simulink model "Automata"  (R2018a)
settings: Solver=VariableStepAuto  StartTime=0.0  StopTime=inf  FixedStep=0.001  RelTol=1e-3
values from neighbouring files (symbols this model uses):
  bcx = 1000e3    (= 1000000)    [Variables.m]
  bcy = 500e3    (= 500000)    [Variables.m]
  beq1 = 30    [Variables.m]
  beq2 = 18    [Variables.m]
  bw = 30000    [Variables.m]
  g = 9.81    [Variables.m]
  Jeq1 = Jwc+Jmc*(rc^2)    (= 2252)    [Variables.m]
  Jeq2 = Jd+Jmi*(riz^2)    (= 27008)    [Variables.m]
  kcy = 1.3e11    (= 130000000000)    [Variables.m]
  Kw = 1800e3    (= 1800000)    [Variables.m]
  Mc = 50000    [Variables.m]
  Mt = Mc+Jeq1*(1/(Rw^2))    (= 59008)    [Variables.m]
  rc = 15    [Variables.m]
  Rd = 0.75    [Variables.m]
  riz = 30    [Variables.m]
  Rw = 0.5    [Variables.m]
  Y_t0 = 45    [Variables.m]
undefined symbols (not defined in the file or in its folder): AlturaInicialBarco, AlturaInicialMuelle, cont_muelle_masa, contenedores, PObjetivo_fijo, PObjetivo_incremental, x_der, x_izq, Y_inf_barco, Y_max, Y_muelle, Y_sb
settings Model: Creator=lauta  LastModifiedBy=lauta
settings SolverCC: AlgebraicLoopSolver=LineSearch

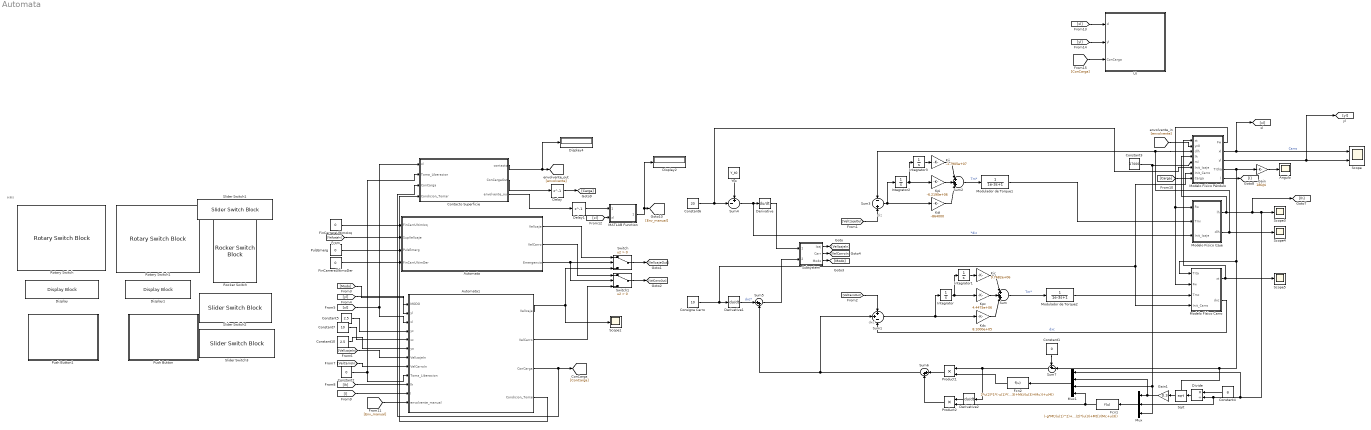
== system Automata ==
  note: HMI
  note: diz
  note: dxc
  Angulo : Scope
  Automata : Stateflow chart  TreatAsAtomicUnit=on
  Automata1 : Stateflow chart  TreatAsAtomicUnit=on
  Consigna Carro : Constant  Value=10
  Constant1 : Constant  Value=0
  Constant10 : Constant  Value=2.5
  Constant2 : Constant  Value=0
  Constant3 : Constant  Value=17000
  Constant4 : Constant  Value=g
  Constant5 : Constant  Value=2.5
  Constant6 : Constant  Value=20
  Constant7 : Constant  Value=10
  Contacto Superficie : Stateflow chart  TreatAsAtomicUnit=on
  Delay : Delay  DelayLength=1  InitialCondition=0
  Delay1 : Delay  DelayLength=1  InitialCondition=0
  Derivative : Derivative
  Derivative1 : Derivative
  Derivative2 : Derivative
  Display : DisplayBlock  WebBlockId=717  LabelPosition=Hide
  Display1 : DisplayBlock  WebBlockId=718  LabelPosition=Hide
  Display2 : Display
  Display4 : Display
  Divide : Product  Inputs=*/
  Fcn1 : Fcn  Expr=(-g*Mt/(u(1)^2)+u(2)*(u(3)+Mt))/(Mc+u(3))
  Fcn2 : Fcn  Expr=2*u(2)*1*(-u(1)*((u(3)+Mt)/(u(3)+Mc))+u(4))
  FinCarreraUltimoDer : Constant  Value=0
  FinCarreraUltimoIzq : Constant  Value=0
  Gain : Gain  Gain=180/pi
  Gain1 : Gain  Gain=0.3
  Integrator{,1..3} (4 alike) : Integrator
  Kdc : Gain  Gain=8.1000e+05
  Kdi : Gain  Gain=-864000
  Kic : Gain  Gain=9.7682e+06
  Kii : Gain  Gain=-1.7905e+07
  Kpc : Gain  Gain=4.4475e+06
  Kpi : Gain  Gain=-6.2190e+06
  MATLAB Function : MATLAB Function  TreatAsAtomicUnit=on
  "Modelo Físico Carro " : Subsystem
  Modelo Físico Izaje : Subsystem
  "Modelo Físico Péndulo " : Subsystem
  Modulador de Torque1 : TransferFcn  Denominator=[1e-3 1]
  Modulador de Torque2 : TransferFcn  Denominator=[1e-3 1]
  Mux : Mux  Inputs=3
  Mux1 : Mux
  Product1 : Product
  Product2 : Product
  PulsEmerg : Constant  Value=0
  Push Button : Subsystem  DialogController=hmiCreateDDGDialog  IsWebBlock=on  mask(MWDashboardBlock){webBlockId=2acad30b-f587-4c91-b113-839cda201c99, webBlockType=pushbutton, ShowInLibBrwoser=on, ShowInitialText=on, HMISrcModelName=Automata}
      mask prompts: webBlockId "WebBlock Id"; webBlockType "WebBlock Type"; HMISrcModelName "Source Model"
      mask help: SimulinkHMI:dialogs:PushButtonDialogDesc
      mask Help: helpview([docroot '/mapfiles/simulink.map'], 'hmi_push_button')
      mask Display:
      | model = bdroot(gcb);
      | if strcmp(get_param(model,'BlockDiagramType'), 'library')
      |     image([(matlabroot) '/toolbox/simulink/hmi/icons/PushButton.png']);
      | end
  Push Button1 : Subsystem  DialogController=hmiCreateDDGDialog  IsWebBlock=on  mask(MWDashboardBlock){webBlockId=d4af1492-9a98-42f0-a069-3443a3c3e2ec, webBlockType=pushbutton, ShowInLibBrwoser=on, ShowInitialText=on, HMISrcModelName=Automata}
      mask prompts: webBlockId "WebBlock Id"; webBlockType "WebBlock Type"; HMISrcModelName "Source Model"
      mask help: SimulinkHMI:dialogs:PushButtonDialogDesc
      mask Help: helpview([docroot '/mapfiles/simulink.map'], 'hmi_push_button')
      mask Display:
      | model = bdroot(gcb);
      | if strcmp(get_param(model,'BlockDiagramType'), 'library')
      |     image([(matlabroot) '/toolbox/simulink/hmi/icons/PushButton.png']);
      | end
  Rocker Switch : RockerSwitchBlock  WebBlockId=682  LabelPosition=Hide
      settings: Values={{'Automatico', 'Manual'}, [-1 1]}
  Rotary Switch : RotarySwitchBlock  WebBlockId=715
      settings: Values={{'High', 'Medium', 'Low', 'OFF', 'Low', 'Medium', 'High'}, [-0.15 -0.05 -0.01 0 0.01 0.05 0.15]}
  Rotary Switch1 : RotarySwitchBlock  WebBlockId=716
      settings: Values={{'High', 'Medium', 'Low', 'OFF', 'Low', 'Medium', 'High'}, [-0.15 -0.05 -0.01 0 0.01 0.05 0.15]}
  Scope : Scope  NumInputPorts=2
  Scope{1,3..5} (4 alike) : Scope
  Slider Switch1 : SliderSwitchBlock  WebBlockId=725
      settings: Values={{'OK', 'STOP'}, [0 1]}
  Slider Switch2 : SliderSwitchBlock  WebBlockId=741
      settings: Values={{'OK', 'LimDerecho'}, [0 1]}
  Slider Switch3 : SliderSwitchBlock  WebBlockId=742
      settings: Values={{'OK', 'LimIzquierdo'}, [0 1]}
  Sqrt : Sqrt  SaturateOnIntegerOverflow=on
  Subsystem : Subsystem
  Sum : Sum  Inputs=|+++|
  Sum1 : Sum  Inputs=++-
  Sum2 : Sum  Inputs=|+++|
  Sum3 : Sum  Inputs=-+
  Sum4 : Sum  Inputs=+-|
  Sum5 : Sum  Inputs=|++
  Sum6 : Sum  Inputs=|++
  Sum7 : Sum  Inputs=+-|
  Switch : Switch  Criteria=u2 > Threshold
  Switch1 : Switch  Criteria=u2 > Threshold
  UI : Stateflow chart  TreatAsAtomicUnit=on
  Yto : Constant  Value=Y_t0
  wires:
  Modelo Físico Izaje/1(lh) -> [lh], Scope3/1, Mux1/1, Divide/2, Mux/2, "Modelo Físico Péndulo "/4(lh)
  Modelo Físico Izaje/2(dlh) -> Scope4/1, "Modelo Físico Péndulo "/3(dlh), Sum3/1
  "Modelo Físico Carro "/1(xt) -> "Modelo Físico Péndulo "/1(xt), Scope5/1
  "Modelo Físico Péndulo "/1(Fw) -> "Modelo Físico Carro "/2(Fw), Modelo Físico Izaje/1(Fw)
  "Modelo Físico Péndulo "/2(xl) -> [xl], Scope/1  "Carro"
  Kpc/1 -> Sum/2
  Sum1/1 -> Kdc/1, Integrator/1
  Integrator/1 -> Kpc/1, Integrator1/1
  Sum/1 -> Modulador de Torque2/1  "Tm*"
  Kdc/1 -> Sum/3
  Integrator1/1 -> Kic/1
  Kic/1 -> Sum/1
  Kii/1 -> Sum2/1
  Integrator3/1 -> Kii/1
  Sum2/1 -> Modulador de Torque1/1  "Tm*"
  Sum3/1 -> Kdi/1, Integrator2/1
  Kdi/1 -> Sum2/3
  Integrator2/1 -> Integrator3/1, Kpi/1
  Kpi/1 -> Sum2/2
  Gain/1 -> Angulo/1
  "Modelo Físico Péndulo "/4(Titha) -> "Modelo Físico Carro "/1(Tita), Sum7/2, Gain/1
  "Modelo Físico Carro "/2(dxc) -> Sum1/3  "dxc"
  Constant3/1 -> Mux/3, Mux1/3, "Modelo Físico Péndulo "/5(ml)
  Modulador de Torque1/1 -> Modelo Físico Izaje/2(Tmi)
  Product1/1 -> Sum6/1
  Product2/1 -> Sum6/2
  Fcn2/1 -> Product1/2
  Fcn1/1 -> Mux1/4, Product2/2
  Sum7/1 -> Product1/1, Derivative2/1
  Derivative2/1 -> Product2/1
  Divide/1 -> Sqrt/1
  Constant4/1 -> Divide/1
  Sqrt/1 -> Gain1/1
  Mux/1 -> Fcn1/1
  Gain1/1 -> Mux1/2, Mux/1
  Mux1/1 -> Fcn2/1
  Constant1/1 -> Sum7/1
  Modulador de Torque2/1 -> "Modelo Físico Carro "/3(Tmc)
  Sum4/1 -> Modelo Físico Izaje/3(Init_Izaje), Derivative/1  "*diz"
  Sum6/1 -> Sum1/2, Sum5/2
  Constant6/1 -> "Modelo Físico Péndulo "/6(Init_Izaje), Sum4/2
  Yto/1 -> Sum4/1
  Consigna Carro/1 -> "Modelo Físico Péndulo "/7(Init_Carro), "Modelo Físico Carro "/4(Init_Carro), Derivative1/1
  Derivative/1 -> Subsystem/1(VelIzaje)
  Derivative1/1 -> Sum5/1  "dxc*"
  Sum5/1 -> Subsystem/2(VelCarro)
  FinCarreraUltimoIzq/1 -> Automata/1(FinCarrUltimIzq)
  [VelIzajeIn] -> Automata/2(SupVelIzaje)
  PulsEmerg/1 -> Automata/3(PulsEmerg)
  FinCarreraUltimoDer/1 -> Automata/4(FinCarrUltimDer)
  Automata/3(Emergencia) -> Switch1/2, Switch/2
  Automata1/1(VelIzaje) -> Scope1/1, Switch/3
  Automata/1(VelIzaje) -> Switch/1
  Automata1/2(VelCarro) -> Switch1/3
  Automata/2(VelCarro) -> Switch1/1
  Subsystem/1(Izaj) -> [VelIzajeIn]
  Switch/1 -> [VelIzajeOut]
  [VelIzajeOut] -> Sum3/2
  [VelCarroOut] -> Sum1/1
  Switch1/1 -> [VelCarroOut]
  Subsystem/3(Modo) -> [Modo]
  [Modo] -> Automata1/1(MODO)
  Subsystem/2(Carr) -> [VelCarroIn]
  [yl] -> Automata1/2(yl)
  [xl] -> Automata1/3(xl), Contacto Superficie/1(xl)
  [VelIzajeIn] -> Automata1/7(VelIzajeIn)
  [VelCarroIn] -> Automata1/8(VelCarroIn)
  Constant2/1 -> Contacto Superficie/2(Toma_Liberacion), Automata1/9(Toma_Liberacion)
  "Modelo Físico Péndulo "/5(l) -> [l]
  [lh] -> Automata1/10(lh)
  [l] -> Automata1/11(l)
  Constant7/1 -> Automata1/5(xc)
  Constant5/1 -> Automata1/4(yc)
  Constant10/1 -> Automata1/6(yo)
  [envolvente] -> "Modelo Físico Péndulo "/2(yc0)
  Automata1/3(ConCarga) -> [ConCarga], Contacto Superficie/3(ConCarga)
  "Modelo Físico Péndulo "/3(yl) -> [yl], Scope/2
  [Carga] -> "Modelo Físico Péndulo "/8(Carga)
  Contacto Superficie/1(contacto) -> Display4/1, [envolvente]
  Contacto Superficie/2(ConCargaOut) -> Delay/1
  Delay/1 -> [Carga]
  Automata1/4(Condicion_Tomar) -> Contacto Superficie/4(Condicion_Tomar)
  Contacto Superficie/3(envolvente_out) -> Delay1/1
  MATLAB Function/1(altura_manual) -> Display2/1, [Env_manual]
  [Env_manual] -> Automata1/12(envolvente_manual)
  Delay1/1 -> MATLAB Function/1(envolventes)
  [xl] -> MATLAB Function/2(xl)
  [xl] -> UI/1(xl)
  [yl] -> UI/2(yl)
  [ConCarga] -> UI/3(ConCarga)

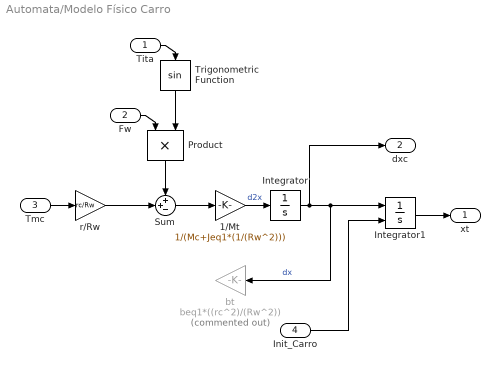
== system Automata/Modelo Físico Carro  ==
  Tita : Inport
  Fw : Inport  Port=2
  Tmc : Inport  Port=3
  Init_Carro : Inport  Port=4
  1/Mt : Gain  Gain=1/(Mc+Jeq1*(1/(Rw^2)))
  Integrator : Integrator
  Integrator1 : Integrator  InitialConditionSource=external
  Product : Product
  Sum : Sum  Inputs=++-
  Trigonometric Function : Trigonometry
  bt : Gain  Commented=on  Gain=beq1*((rc^2)/(Rw^2))
  "r/Rw " : Gain  Gain=rc/Rw
  xt : Outport
  dxc : Outport  Port=2
  wires:
  Tita/1 -> Trigonometric Function/1
  Integrator/1 -> dxc/1, bt/1, Integrator1/1  "dx"
  Product/1 -> Sum/1
  "r/Rw "/1 -> Sum/2
  Sum/1 -> 1/Mt/1
  Trigonometric Function/1 -> Product/2
  Integrator1/1 -> xt/1
  1/Mt/1 -> Integrator/1  "d2x"
  Tmc/1 -> "r/Rw "/1
  Fw/1 -> Product/1
  Init_Carro/1 -> Integrator1/2

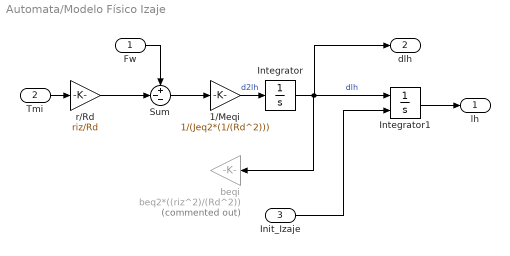
== system Automata/Modelo Físico Izaje ==
  Fw : Inport
  Tmi : Inport  Port=2
  Init_Izaje : Inport  Port=3
  1/Meqi : Gain  Gain=1/(Jeq2*(1/(Rd^2)))
  Integrator : Integrator
  Integrator1 : Integrator  InitialConditionSource=external
  Sum : Sum  Inputs=+--
  beqi : Gain  Commented=on  Gain=beq2*((riz^2)/(Rd^2))
  "r/Rd " : Gain  Gain=riz/Rd
  lh : Outport
  dlh : Outport  Port=2
  wires:
  "r/Rd "/1 -> Sum/2
  Sum/1 -> 1/Meqi/1
  Integrator/1 -> beqi/1, dlh/1, Integrator1/1  "dlh"
  Tmi/1 -> "r/Rd "/1
  Integrator1/1 -> lh/1
  1/Meqi/1 -> Integrator/1  "d2lh"
  Fw/1 -> Sum/1
  Init_Izaje/1 -> Integrator1/2

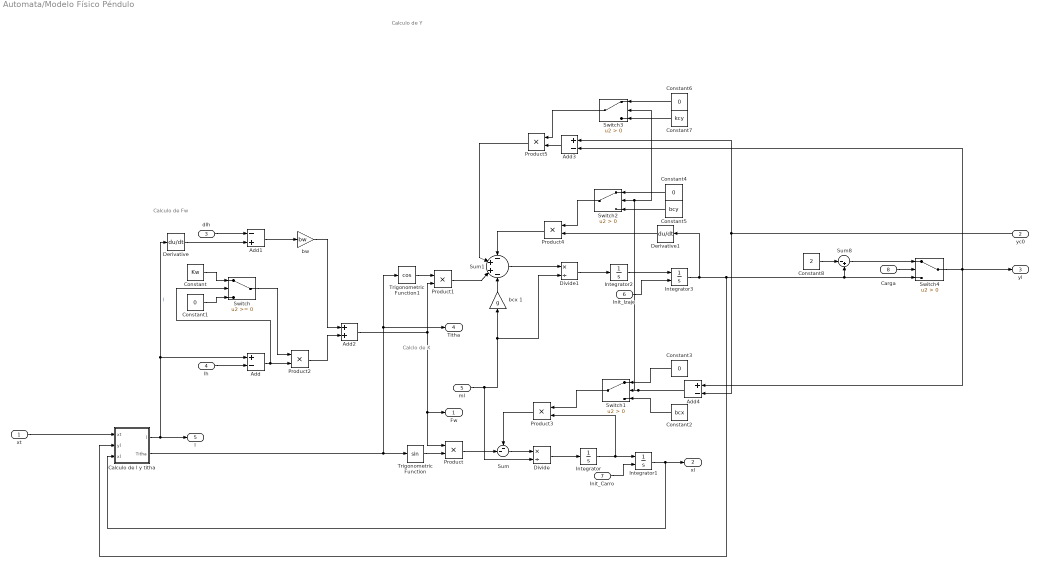
== system Automata/Modelo Físico Péndulo  ==
  note: Calculo de Fw
  note: Calclo de X
  note: Calculo de Y
  xt : Inport
  yc0 : Inport  Port=2
  dlh : Inport  Port=3
  lh : Inport  Port=4
  ml : Inport  Port=5
  Init_Izaje : Inport  Port=6
  Init_Carro : Inport  Port=7
  Carga : Inport  Port=8
  Add : Sum  Inputs=+-
  Add1 : Sum  Inputs=-+
  Add2 : Sum
  Add3 : Sum  Inputs=+-
  Add4 : Sum  Inputs=+-
  Calculo de l y titha : Subsystem
  Constant : Constant  Value=Kw
  Constant{1,3..4,6} (4 alike) : Constant  Value=0
  Constant2 : Constant  Value=bcx
  Constant5 : Constant  Value=bcy
  Constant7 : Constant  Value=kcy
  Constant8 : Constant  Value=2
  Derivative : Derivative
  Derivative1 : Derivative
  Divide : Product  Inputs=*/
  Divide1 : Product  Inputs=*/
  Integrator : Integrator
  Integrator1 : Integrator  InitialConditionSource=external
  Integrator2 : Integrator
  Integrator3 : Integrator  InitialConditionSource=external  InitialCondition=20
  Product{,1..5} (6 alike) : Product
  Sum : Sum  Inputs=--|
  Sum1 : Sum  Inputs=-|+|+|-
  Sum8 : Sum  Inputs=|-+
  Switch : Switch
  Switch{1..4} (4 alike) : Switch  Criteria=u2 > Threshold
  Trigonometric Function : Trigonometry
  Trigonometric Function1 : Trigonometry  Operator=cos
  bcx 1 : Gain  Gain=g
  bw : Gain  Gain=bw
  Fw : Outport
  xl : Outport  Port=2
  yl : Outport  Port=3
  Titha : Outport  Port=4
  l : Outport  Port=5
  wires:
  xt/1 -> Calculo de l y titha/1(xt)
  Calculo de l y titha/1(l) -> Add/1, Derivative/1, l/1  "l"
  lh/1 -> Add/2
  Add/1 -> Switch/2, Product2/2
  Add1/1 -> bw/1
  Product2/1 -> Add2/2
  bw/1 -> Add2/1
  dlh/1 -> Add1/1
  Derivative/1 -> Add1/2
  Add2/1 -> Fw/1, Product/1, Product1/2
  Trigonometric Function/1 -> Product/2
  Calculo de l y titha/2(Titha) -> Titha/1, Trigonometric Function1/1, Trigonometric Function/1
  Product/1 -> Sum/2
  Sum/1 -> Divide/1
  Integrator/1 -> Product3/2, Integrator1/1
  Product3/1 -> Sum/1
  Integrator1/1 -> xl/1, Calculo de l y titha/3(xl)
  Trigonometric Function1/1 -> Product1/1
  ml/1 -> Divide1/2, bcx 1/1, Divide/2
  Divide/1 -> Integrator/1
  Product1/1 -> Sum1/3
  bcx 1/1 -> Sum1/4
  yc0/1 -> Add3/1, Add4/2
  Product5/1 -> Sum1/2
  Product4/1 -> Sum1/1
  Integrator2/1 -> Integrator3/1
  Sum1/1 -> Divide1/1
  Divide1/1 -> Integrator2/1
  Switch/1 -> Product2/1
  Constant/1 -> Switch/1
  Constant1/1 -> Switch/3
  Switch1/1 -> Product3/1
  Add4/1 -> Switch3/2, Switch2/2, Switch1/2
  Constant3/1 -> Switch1/1
  Constant2/1 -> Switch1/3
  Switch2/1 -> Product4/1
  Constant4/1 -> Switch2/1
  Constant5/1 -> Switch2/3
  Add3/1 -> Product5/2
  Switch3/1 -> Product5/1
  Constant6/1 -> Switch3/1
  Constant7/1 -> Switch3/3
  Derivative1/1 -> Product4/2
  Init_Carro/1 -> Integrator1/2
  Init_Izaje/1 -> Integrator3/2
  Switch4/1 -> Add3/2, Add4/1, yl/1
  Constant8/1 -> Sum8/1
  Sum8/1 -> Switch4/1
  Carga/1 -> Switch4/2
  Integrator3/1 -> Calculo de l y titha/2(yl), Switch4/3, Sum8/2, Derivative1/1

== system Automata/Push Button ==

== system Automata/Push Button1 ==

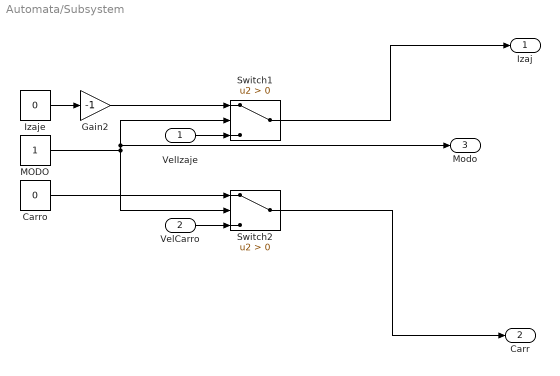
== system Automata/Subsystem ==
  VelIzaje : Inport
  VelCarro : Inport  Port=2
  Carro : Constant  Value=0
  Gain2 : Gain  Gain=-1
  Izaje : Constant  Value=0
  MODO : Constant
  Switch1 : Switch  Criteria=u2 > Threshold
  Switch2 : Switch  Criteria=u2 > Threshold
  Izaj : Outport
  Carr : Outport  Port=2
  Modo : Outport  Port=3
  wires:
  Gain2/1 -> Switch1/1
  Izaje/1 -> Gain2/1
  Switch1/1 -> Izaj/1
  MODO/1 -> Modo/1, Switch1/2, Switch2/2
  Carro/1 -> Switch2/1
  Switch2/1 -> Carr/1
  VelIzaje/1 -> Switch1/3
  VelCarro/1 -> Switch2/3

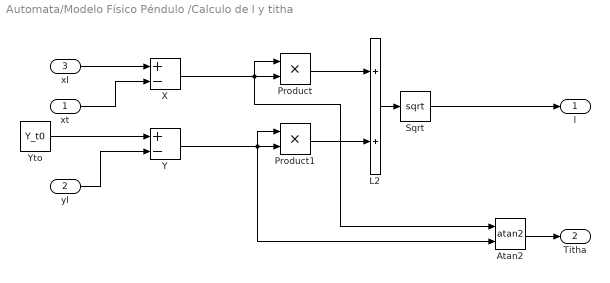
== system Automata/Modelo Físico Péndulo /Calculo de l y titha ==
  xt : Inport
  yl : Inport  Port=2
  xl : Inport  Port=3
  Atan2 : Trigonometry  Operator=atan2
  L2 : Sum
  Product : Product
  Product1 : Product
  Sqrt : Sqrt  SaturateOnIntegerOverflow=on
  X : Sum  Inputs=+-
  Y : Sum  Inputs=+-
  Yto : Constant  Value=Y_t0
  l : Outport
  Titha : Outport  Port=2
  wires:
  Y/1 -> Atan2/2, Product1/1, Product1/2
  X/1 -> Product/2, Atan2/1, Product/1
  Product1/1 -> L2/2
  L2/1 -> Sqrt/1
  yl/1 -> Y/2
  Product/1 -> L2/1
  Yto/1 -> Y/1
  xl/1 -> X/1
  Sqrt/1 -> l/1
  xt/1 -> X/2
  Atan2/1 -> Titha/1

== stateflow chart Automata/Automata ==
  state NIVEL_0
    if PulsEmerg==1 || FinCarrUltimDer==1 || FinCarrUltimIzq==1 || SupVelIzaje>10
    VelIzaje=0;
    VelCarro=0;
    Emergencia=1;
    else
    Emergencia=-1;
    end
  (default) -> NIVEL_0
  data: FinCarrUltimIzq input; SupVelIzaje input; PulsEmerg input; FinCarrUltimDer input; VelIzaje output; VelCarro output; Emergencia output

== stateflow chart Automata/Automata1 ==
  state NIVEL_1
    contenedores;
    cont_muelle_masa;
    entry: ConCarga=-1;
    note: -Comando operador
        | -Limites normales de oepracion
        | 	-Activacion/desactivacion de control de angulo
        | 	-Fines de carrera
        | 	-Control de Velocidad
        | 	-Estado de carga
        | 		-4 Sensores
        | 		-Twistlook
        | 	-Deteccion cable de izaje flojo
        | 	-Sensor de angulo
    state MODOS [parallel]
      settings: executionOrder=1
      state MANUAL
        state Liberacion
          Condicion_Tomar=-1;
          if Toma_Liberacion==-1
          ConCarga=-1;
          end
        state Toma
          Condicion_Tomar=1;
          if Toma_Liberacion==1
          ConCarga=1;
          end
        state Aproximacion
          Condicion_Tomar=0;
          VelCarro=VelCarroIn*0.1;
          VelIzaje=VelIzajeIn*0.1;
        note: -Falta asignar yc = y consigna
            | -Falta asignar xc = x consigna
        (junction 70) -> Toma [order 1] : [ConCarga==-1]
        (junction 70) -> Liberacion [order 2] : [ConCarga==1]
        Aproximacion -> (junction 70) : [yl==yc && xl<xc+0.1 && xl>xc-0.1]
        (default) -> Aproximacion
        Toma -> Aproximacion : [ConCarga==1]
        Liberacion -> Aproximacion : [ConCarga==-1]
      note: -Falta asignar yo como yc anterior
      state AUTOMATICO
        state CONFIGURACION
          x_izq;
          x_der;
          PObjetivo_incremental;
          PObjetivo_fijo;
          Y_inf_barco;
          Y_muelle;
          Y_t0;
          Y_max;
          Y_sb;
          AlturaInicialMuelle;
          AlturaInicialBarco;
        state CICLOS
          VelIzaje=VelIzajeIn;
          VelCarro=VelCarroIn;
          note: -Toma de carga (M) OK
              | -Izaje y traslacion (A)
              | -Parada y descenso (A)
              | -Aproximacion fina (M) OK
              | -Liberacion de carga (M) OK
              | -Retorno vacio (A)
        (default) -> CONFIGURACION
        CONFIGURACION -> CICLOS
      (default) -> MANUAL
      MANUAL -> AUTOMATICO : [((yl>(yo+2.5))  &&xl<0) || ((yl>(yo+2.5)) && xl>5)]
      AUTOMATICO -> MANUAL : [((yl<(yc+2.5) && xl<xc+0.1 && xl>xc-0.1) && xl<0) || ((yl<(yc+2.5) && xl<xc+0.1 && xl>xc-0.1) && xl>5)]
  (default) -> NIVEL_1
  data: VelIzaje output; VelCarro output; MODO input; yl input; Y_inf_barco parameter; AlturaInicialBarco parameter; AlturaInicialMuelle parameter; PObjetivo_fijo parameter; PObjetivo_incremental parameter; x_izq parameter; x_der parameter; Y_muelle parameter; Y_t0 parameter; Y_max parameter; Y_sb parameter; xl input; yc input; xc input; yo input; VelIzajeIn input; VelCarroIn input; Toma_Liberacion input; lh input; l input; CargaDescarga local =0; cont_muelle_masa parameter; contenedores parameter; ConCarga output; Condicion_Tomar output; envolvente_manual input

== stateflow chart Automata/Contacto Superficie ==
  state ModeloContacto
    envolvente;
    entry: envolventes=envolvente;
    envolvente_out=envolventes;
    state ContactoConstante [parallel]
      contacto=envolventes(2,round((30+xl)/0.5)+1);
      ConCargaOut=ConCarga;
      settings: executionOrder=2
    state ContactoActualizacion [parallel]
      if Toma_Liberacion==1 && Condicion_Tomar==1
      index=round((30+xl)/0.5)+1;
      if envolventes(1,index)<=xl
      for i=1:5
      envolventes(2,index-3+i)=envolventes(2,index-3+i)-2.5;
      end
      elseif envolventes(1,index)>xl
      for i=1:5
      envolventes(2,index-4+i)=envolventes(2,index-4+i)-2.5;
      end
      end
      elseif Toma_Liberacion==-1 && Condicion_Tomar==1
      index=round((30+xl)/0.5)+1;
      if envolventes(1,index)<=xl
      for i=1:5
      envolventes(2,index-3+i)=envolventes(2,index-3+i)+2.5;
      end
      elseif envolventes(1,index)>xl
      for i=1:5
      envolventes(2,index-4+i)=envolventes(2,index-4+i)+2.5;
      end
      end
      end
      settings: executionOrder=1
  data: envolvente parameter; xl input; contacto output; envolventes local; Toma_Liberacion input; i local; index local; ConCarga input; ConCargaOut output; Condicion_Tomar input; envolvente_out output

== matlab function Automata/MATLAB Function ==
  data: envolventes input; altura_manual output; xl input
function altura_manual = env(envolventes,xl)
altura_manual=zeros(1,1);
envolvente_manual=zeros(2,161);

x=envolventes(1,:);
y=envolventes(2,:);
xnuevo=x;
ynuevo=y;

for i=71:5:length(x)
    if i==71
        if ((y(i-1)-y(i))>2.5 || (y(i+5)-y(i))>2.5)
            aux=max(y(i-1),y(i+5));
            for j=0:4
                ynuevo(i+j)=aux;
            end
        end
        
    else
        
        if i~=length(x) && (y(i-5)-y(i)>2.5 || y(i+5)-y(i)>2.5)
            aux=max(y(i-5),y(i+5));
            for j=0:4
                ynuevo(i+j)=aux;
            end
        else
            if i~=length(x)
                for j=0:4
                    ynuevo(i+j)=y(i);
                end
            else
                ynuevo(i)=y(i);
            end
        end
    end
end
for i=71:length(xnuevo)
    ynuevo(i)=ynuevo(i)+2.5;
end
envolvente_manual(1,:)=xnuevo;
envolvente_manual(2,:)=ynuevo;
altura_manual=envolvente_manual(2,round((30+xl)/0.5)+1);
end

== stateflow chart Automata/UI ==
  state Graficador
    en: coder.extrinsic('Automatas', 'actualizarPosiciones')
    app = Automatas();
    during: actualizarPosiciones(app,xl,yl,ConCarga);
  (default) -> Graficador
  data: app local; xl input; yl input; ConCarga input
